simulink model "tennode_3"  (R2018b)
settings: Solver=ode3  StartTime=0.0  StopTime=5  FixedStep=Ts  RelTol=1e-3
values from neighbouring files (symbols this model uses):
  BESS_mode = 0    [load_vars.m]
  line1 = line1_length*R1    (= 0.01273)    [load_vars.m]
  line10 = line10_length*R1    (= 0.01273)    [load_vars.m]
  LINE10_en = 1    [load_vars.m]
  line11 = line11_length*R1    (= 0.01273)    [load_vars.m]
  LINE11_en = 1    [load_vars.m]
  line12 = line12_length*R1    (= 0.02546)    [load_vars.m]
  LINE12_en = 1    [load_vars.m]
  line13 = line13_length*R1    (= 0.015276)    [load_vars.m]
  LINE13_en = 1    [load_vars.m]
  line14 = line14_length*R1    (= 0.019095)    [load_vars.m]
  LINE14_en = 1    [load_vars.m]
  line15 = line15_length*R1    (= 0.014003)    [load_vars.m]
  LINE15_en = 1    [load_vars.m]
  line16 = line16_length*R1    (= 0.034371)    [load_vars.m]
  LINE16_en = 1    [load_vars.m]
  line17 = line17_length*R1    (= 0.017822)    [load_vars.m]
  LINE17_en = 1    [load_vars.m]
  LINE1_en = 1    [load_vars.m]
  line2 = line2_length*R1    (= 0.02546)    [load_vars.m]
  LINE2_en = 1    [load_vars.m]
  line3 = line3_length*R1    (= 0.015276)    [load_vars.m]
  LINE3_en = 1    [load_vars.m]
  line4 = line4_length*R1    (= 0.019095)    [load_vars.m]
  LINE4_en = 1    [load_vars.m]
  line5 = line5_length*R1    (= 0.014003)    [load_vars.m]
  LINE5_en = 1    [load_vars.m]
  line6 = line6_length*R1    (= 0.01273)    [load_vars.m]
  LINE6_en = 1    [load_vars.m]
  line7 = line7_length*R1    (= 0.03819)    [load_vars.m]
  LINE7_en = 1    [load_vars.m]
  line8 = line8_length*R1    (= 0.01273)    [load_vars.m]
  LINE8_en = 1    [load_vars.m]
  line9 = line9_length*R1    (= 0.01273)    [load_vars.m]
  LINE9_en = 1    [load_vars.m]
  t_contingency = 1    [load_vars.m]
  Ts = 0.0001    [load_vars.m]
  uDemand1 = 20e3    (= 20000)    [load_vars.m]
  uDemand10 = 20e3    (= 20000)    [load_vars.m]
  uDemand2 = 20e3    (= 20000)    [load_vars.m]
  uDemand3 = 20e3    (= 20000)    [load_vars.m]
  uDemand4 = 20e3    (= 20000)    [load_vars.m]
  uDemand5 = 20e3    (= 20000)    [load_vars.m]
  uDemand6 = 20e3    (= 20000)    [load_vars.m]
  uDemand7 = 20e3    (= 20000)    [load_vars.m]
  uDemand8 = 20e3    (= 20000)    [load_vars.m]
  uDemand9 = 20e3    (= 20000)    [load_vars.m]
undefined symbols (not defined in the file or in its folder): DER10_BESS_en, DER1_BESS_en, DER2_BESS_en, DER3_BESS_en, DER4_BESS_en, DER5_BESS_en, DER6_BESS_en, DER7_BESS_en, DER8_BESS_en, DER9_BESS_en, DR_capacity_1, DR_capacity_10, DR_capacity_2, DR_capacity_3, DR_capacity_4, DR_capacity_5, DR_capacity_6, DR_capacity_7, DR_capacity_8, DR_capacity_9, P_set1, P_set10, P_set2, P_set3, P_set4, P_set5, P_set6, P_set7, P_set8, P_set9, PV_capacity_1, PV_capacity_10, PV_capacity_2, PV_capacity_3, PV_capacity_4, PV_capacity_5, PV_capacity_6, PV_capacity_7, PV_capacity_8, PV_capacity_9, PV_en_1, PV_en_10, PV_en_2, PV_en_3, PV_en_4, PV_en_5, PV_en_6, PV_en_7, PV_en_8, PV_en_9
libraries: powerlib x232, simulink x66, powerlib_meascontrol x23, sps_avr x1, spsDieselMotorModel x1
(part 1 of 7)
settings Model: Creator=jjcla  LastModifiedBy=jjcla
settings SolverCC: ConcurrentTasks=on  AutoInsertRateTranBlk=on

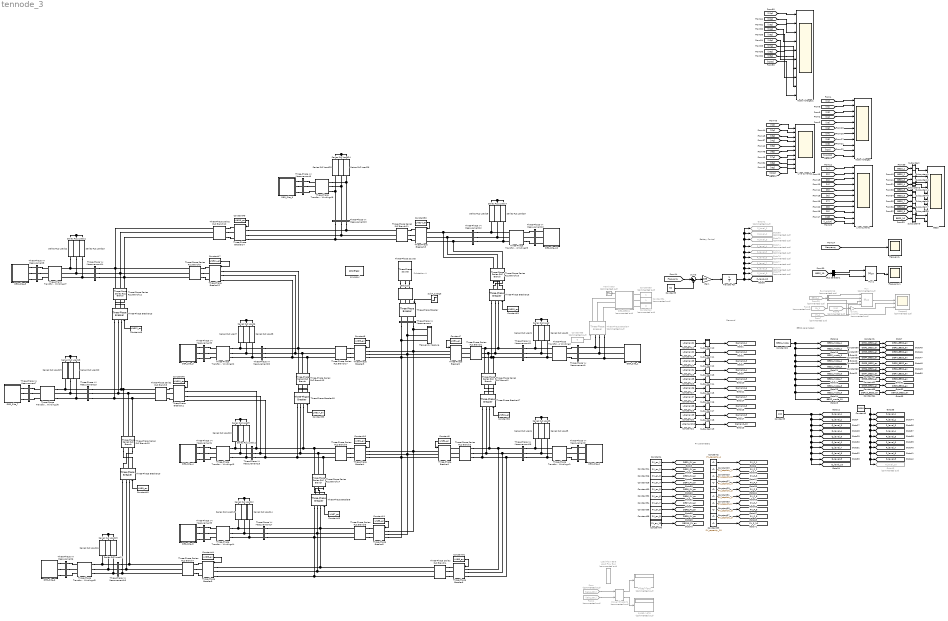
== system tennode_3 ==
  note: Substation A
  note: Battery Control
  note: Demand
  note: BESS parameters
  note: PV parameters
  66k/22k : powerlib/Elements/Three-Phase Transformer (Two Windings)  Winding1Connection=Yg  Winding2Connection=Y  CoreType=Three single-phase transformers  SetSaturation=off  Hysteresis=off  DataFile='hysteresis'  SetInitialFlux=off  Measurements=None  UNITS=pu  NominalPower=[ 10e6 , 50 ]  Winding1=[ 66e3 , 0.002 , 0.08 ]  Winding2=[22e3 , 0.002 , 0.08 ]  Rm=500  Lm=500  L0=0.5  Saturation=[ 0,0 ; 0.0024,1.2 ; 1.0,1.52 ]  InitialFluxes=[ 0.8 , -0.8 , 0.7 ]  MoreParameters=off  BreakLoop=on  DataType=off  TransfoNumber=1
      settings: SourceProductName=Simscape Electrical
  BESS : Scope  NumInputPorts=10
  Bus Selector1 : BusSelector  OutputSignals=Pbatt,Qbatt
  Bus Selector16 : BusSelector  Commented=on  OutputSignals=Pbatt,Qbatt,SOC (%)
  Constant1 : Constant  Value=DER1_BESS_en
  Constant10 : Constant  Value=LINE4_en
  Constant11 : Constant  Value=LINE5_en
  Constant12 : Constant  Value=uDemand1
  Constant13 : Constant  Value=uDemand2
  Constant14 : Constant  Value=uDemand3
  Constant15 : Constant  Value=uDemand4
  Constant16 : Constant  Value=uDemand5
  Constant17 : Constant  Value=uDemand6
  Constant18 : Constant  Value=uDemand7
  Constant19 : Constant  Value=uDemand8
  Constant2 : Constant  Value=PV_capacity_1
  Constant20 : Constant  Value=uDemand9
  Constant21 : Constant  Value=uDemand10
  Constant22 : Constant  Value=BESS_mode
  Constant23 : Constant  Value=PV_capacity_2
  Constant24 : Constant  Value=PV_en_2
  Constant25 : Constant  Value=PV_capacity_3
  Constant26 : Constant  Value=PV_en_3
  Constant27 : Constant  Value=PV_capacity_4
  Constant28 : Constant  Value=PV_en_4
  Constant29 : Constant  Value=PV_capacity_5
  Constant3 : Constant  Value=LINE2_en
  Constant30 : Constant  Value=PV_en_5
  Constant31 : Constant  Value=PV_capacity_6
  Constant32 : Constant  Value=PV_en_6
  Constant33 : Constant  Value=PV_capacity_7
  Constant34 : Constant  Value=PV_en_7
  Constant35 : Constant  Value=PV_capacity_8
  Constant36 : Constant  Value=PV_en_8
  Constant37 : Constant  Value=PV_capacity_9
  Constant38 : Constant  Value=PV_en_9
  Constant39 : Constant  Value=PV_capacity_10
  Constant4 : Constant  Value=PV_en_1
  Constant40 : Constant  Value=PV_en_10
  Constant41 : Constant  Value=LINE6_en
  Constant42 : Constant  Commented=on  Value=0
  Constant43 : Constant  Value=LINE7_en
  Constant44 : Constant  Value=LINE8_en
  Constant45 : Constant  Value=LINE9_en
  Constant46 : Constant  Value=LINE10_en
  Constant47 : Constant  Value=LINE11_en
  Constant48 : Constant  Value=LINE12_en
  Constant49 : Constant  Value=LINE13_en
  Constant5 : Constant  Value=100
  Constant50 : Constant  Value=LINE14_en
  Constant51 : Constant  Value=LINE15_en
  Constant52 : Constant  Value=LINE16_en
  Constant53 : Constant  Value=LINE17_en
  Constant54 : Constant  Commented=on
  Constant55 : Constant  Commented=on
  Constant56 : Constant  Value=DER2_BESS_en
  Constant57 : Constant  Value=DER3_BESS_en
  Constant58 : Constant  Value=DER4_BESS_en
  Constant59 : Constant  Value=DER5_BESS_en
  Constant6 : Constant  Value=5000
  Constant60 : Constant  Value=DER6_BESS_en
  Constant61 : Constant  Value=DER7_BESS_en
  Constant62 : Constant  Value=DER8_BESS_en
  Constant63 : Constant  Value=DER9_BESS_en
  Constant64 : Constant  Value=DER10_BESS_en
  Constant65 : Constant  Commented=on  Value=0
  Constant7 : Constant  Value=LINE1_en
  Constant8 : Constant  Value=LINE3_en
  Constant9 : Constant  Value=50
  DER_BESS1 : Subsystem  Commented=on  AncestorBlock=|  mask(Grid-connected Energy Storage (PQ Model)){SimMode=Electromagnetic Transient (EMT), Vn=400, Fn=50, PnomkW=5, kWh_Rated=13.5, Efficiency=96, LimitVec=[90 10], RechargeSOC=90, Precharge=50, autoRecharge=on, Initial_kWh_pc=80, PQvec=[500e3 0]}
      | microgridLibrary1/Energy Storage
      | (PQ Model)
      mask prompts: SimMode "Simulation Mode"; Vn "Nominal L-L Voltage [Vrms]"; Fn "Nominal Frequency [Hz]"; PnomkW "Rated Power [kW]"; kWh_Rated "Rated Capacity [kWh]"; Efficiency "Overall System Efficiency [%]"; LimitVec "Upper/Lower Charge Limits [%]"; RechargeSOC "SOC to Recharge [%]"; Precharge "Recharge Rate [% of Rated Power]"; autoRecharge "Enable Auto-Recharge"; Initial_kWh_pc "Initial State-of-Charge [0-100%]"; PQvec "Initial Active/Reactive Cmds"
      mask help:
      | The energy storage block models a generic grid-connected energy storage system (ESS), most commonly a battery system. This is a system-level model that does not contain any power electronics, but is useful for load flow, phasor, and hybrid phasor-EMT simulations. The inputs to this block are the commanded active and reactive power of the ESS. The ESS is assumed to have four quadrent operation. The Mode Input dictates what high-level operation the ESS has: current control (Mode = 1) or voltage control (Mode = 0). Current control is ideal for a grid connected system where you need to specify P,Q commands. Voltage control is necessary if the ESS will be the only system supporting the microgrid in islanded mode.
      |
      | For more detailed ESS models, consider the battery block in the Drives library. Consider using this PQ Model to perform load flow studies and switch to a more detailed model when full EMT studies or more advanced controls are required.
      |
      | Note: The initial active/reactive power commands must be specified for use for Load Flow analysis.
      mask init:
      | % Calculate Initial Conditions
      | Pnom = PnomkW*1e3;
      | P0 = -PQvec(1);  Q0 = -PQvec(2);
      | if abs(P0) > Pnom
      |     P0 = sign(P0)*Pnom;
      | end
      | 
      | % Calculate Q0 given Reactive Power Capability Curve
      | Qlim = sqrt(Pnom^2 - P0^2);
      | if Qlim > abs(Q0)
      |     Q0 = sign(Q0)*Qlim;
      | end
      | 
      | UpChrgLim = LimitVec(1);
      | LowChrgLim = LimitVec(2);
      | if Initial_kWh_pc > UpChrgLim && P0 < 0
      |     P0 = 0; Q0 = 0;
      | elseif Initial_kWh_pc < LowChrgLim && P0 > 0
      |     P0 = 0; Q0 = 0;
      | end
      | 
      | simulationStatus =  get_param(bdroot,'SimulationStatus');
      | 
      | % The active variant can only be modified at edit-time or very early during
      | % the simulink compile stage. 
      | if any(strcmp(simulationStatus, {'stopped'}))
      | 
      | blk = [gcb '/Power Measures'];
      | if strcmp(SimMode,'Phasor')
      |     set_param(blk,'OverrideUsingVariant','Phasor');
      | else
      |     set_param(blk,'OverrideUsingVariant','EMT');
      | end
      | 
      | 
      | end
      mask TypeOptions SimMode: Electromagnetic Transient (EMT) | Phasor
      mask DialogControl Container7 Prompt: Grid Connection Properties
      mask DialogControl Container11 Prompt: Charge/Discharge Controls
      mask DialogControl Container12 Prompt: Initial Conditions
      mask Display: plot(-80,-50,80,50,[0,9,18,24,29,30,29,24,18,9,0,-9,-18,-24,-29,-30,-29,-24,-18,-9,0],[30,29,24,18,9,0,-9,-18,-24,-29,-30,-29,-24,-18,-9,0,9,18,24,29,30],[-50],[0],[50],[0],[45 35 40 40 40],[15 15 15 20 10],[1 2 3 4 5 6 7 8 9 10 11 12 13 14 15 16 17 18 19 20 21].*1.5-15,[0,9,18,24,29,30,29,24,18,9,0,-9,-18,-24,-29,-30,-29,-24,-18,-9,0]./2.4)
  DER_Site_1 : Subsystem
  DER_Site_10 : Subsystem
  DER_Site_2 : Subsystem
  DER_Site_3 : Subsystem
  DER_Site_4 : Subsystem
  DER_Site_5 : Subsystem
  DER_Site_6 : Subsystem
  DER_Site_7 : Subsystem
  DER_Site_8 : Subsystem
  DER_Site_9 : Subsystem
  Frequency : Scope
  Frequency Measure : Subsystem
  Frequency1 : Scope
  From : From  Commented=on  GotoTag=Vabc_001  TagVisibility=global
  From1 : From  Commented=on  GotoTag=Iabc_001  TagVisibility=global
  From25 : From  Commented=on  GotoTag=BESS_1  TagVisibility=global
  From6 : From  Commented=on  GotoTag=V1  TagVisibility=global
  From7 : From  Commented=on  GotoTag=PV_1  TagVisibility=global
  From8 : From  Commented=on  GotoTag=SL_1  TagVisibility=global
  Gain : Gain  Gain=1e5
  Goto43 : Goto  Commented=on  GotoTag=P_level_10  TagVisibility=global
  Goto72 : Goto  Commented=on  GotoTag=P_level_1  TagVisibility=global
  Goto73 : Goto  Commented=on  GotoTag=P_level_3  TagVisibility=global
  Goto74 : Goto  Commented=on  GotoTag=P_level_4  TagVisibility=global
  Goto75 : Goto  Commented=on  GotoTag=P_level_5  TagVisibility=global
  Goto76 : Goto  Commented=on  GotoTag=P_level_6  TagVisibility=global
  Goto77 : Goto  Commented=on  GotoTag=P_level_7  TagVisibility=global
  Goto78 : Goto  Commented=on  GotoTag=P_level_8  TagVisibility=global
  Goto79 : Goto  Commented=on  GotoTag=P_level_9  TagVisibility=global
  Goto80 : Goto  Commented=on  GotoTag=P_level_2  TagVisibility=global
  Line Currents : Scope  NumInputPorts=11
  Line Currents1 : Scope  NumInputPorts=10
  Load Flow Bar6 : powerlib/Measurements/Load Flow Bus  Commented=on  LConnTagsString=a|b|c  RConnTagsString=a|b|c  Phases=ABC  Connectors=on both sides  ID=001  Vbase=22000/sqrt(3)  Vref=[1.0 1.0 1.0]  Vangle=[0 -120 120]  VLF=0.9871  VLFb=1.052  VLFc=0.978  angleLF=-5.528  angleLFb=-122.4  angleLFc=116
      settings: AttributesFormatString=%<ID>  SourceProductName=Simscape Electrical
  Mux : Mux  Commented=on
      settings: DisplayOption=signals
  Mux1 : Mux  Inputs=2
      settings: DisplayOption=signals
  Node Voltages : Scope  NumInputPorts=11
  Node Voltages1 : Scope  NumInputPorts=10
  P 692->675 : Display  Commented=on
  Power (Phasor)1 : powerlib_meascontrol/Measurements/Power (Phasor)  Commented=on
      settings: SourceProductName=Simscape Electrical  SourceProductBaseCode=PS
  Q 692->675 : Display  Commented=on
  Scopes1 : Scope  Commented=on  NumInputPorts=4
  Series RLC Load{,1..29} (30 alike) : powerlib/Elements/Series RLC Load  LConnTagsString=a  RConnTagsString=__new0  NominalVoltage=22e3  NominalFrequency=50  ActivePower=10e3  InductivePower=100  CapacitivePower=100  Setx0=off  InitialVoltage=0  SetiL0=off  InitialCurrent=0  Measurements=None  LoadType=constant Z
      settings: SourceProductName=Simscape Electrical
  SubA_outage : Step  Time=t_contingency  Before=1  After=0  SampleTime=0
  Subsystem : Subsystem
  Subsystem1 : Subsystem
  Subsystem10 : Subsystem
  Subsystem11 : Subsystem
  Subsystem12 : Subsystem
  Subsystem13 : Subsystem
  Subsystem14 : Subsystem
  Subsystem15 : Subsystem
  Subsystem16 : Subsystem
  Subsystem17 : Subsystem
  Subsystem18 : Subsystem
  Subsystem19 : Subsystem
  Subsystem2 : Subsystem
  Subsystem3 : Subsystem
  Subsystem4 : Subsystem
  Subsystem5 : Subsystem
  Subsystem6 : Subsystem
  Subsystem7 : Subsystem
  Subsystem8 : Subsystem
  Subsystem9 : Subsystem
  Sum3 : Sum  Inputs=|+-
  Terminator : Terminator  Commented=on
  Three-Phase Series RLC Branch1 : powerlib/Elements/Three-Phase Series RLC Branch  LConnTagsString=A|B|C  RConnTagsString=A|B|C  BranchType=R  Resistance=line1  Inductance=10e-6  Capacitance=10e-9  Measurements=Branch currents
  Three-Phase Series RLC Branch10 : powerlib/Elements/Three-Phase Series RLC Branch  LConnTagsString=A|B|C  RConnTagsString=A|B|C  BranchType=R  Resistance=line13  Inductance=10e-6  Capacitance=10e-9  Measurements=Branch currents
  Three-Phase Series RLC Branch11 : powerlib/Elements/Three-Phase Series RLC Branch  LConnTagsString=A|B|C  RConnTagsString=A|B|C  BranchType=R  Resistance=line14  Inductance=10e-6  Capacitance=10e-9  Measurements=Branch currents
  Three-Phase Series RLC Branch12 : powerlib/Elements/Three-Phase Series RLC Branch  LConnTagsString=A|B|C  RConnTagsString=A|B|C  BranchType=R  Resistance=line12  Inductance=10e-6  Capacitance=10e-9  Measurements=Branch currents
  Three-Phase Series RLC Branch13 : powerlib/Elements/Three-Phase Series RLC Branch  LConnTagsString=A|B|C  RConnTagsString=A|B|C  BranchType=R  Resistance=line17  Inductance=10e-6  Capacitance=10e-9  Measurements=Branch currents
  Three-Phase Series RLC Branch14 : powerlib/Elements/Three-Phase Series RLC Branch  LConnTagsString=A|B|C  RConnTagsString=A|B|C  BranchType=R  Resistance=line7  Inductance=10e-6  Capacitance=10e-9  Measurements=Branch currents
  Three-Phase Series RLC Branch15 : powerlib/Elements/Three-Phase Series RLC Branch  LConnTagsString=A|B|C  RConnTagsString=A|B|C  BranchType=R  Resistance=line9  Inductance=10e-6  Capacitance=10e-9  Measurements=Branch currents
  Three-Phase Series RLC Branch16 : powerlib/Elements/Three-Phase Series RLC Branch  LConnTagsString=A|B|C  RConnTagsString=A|B|C  BranchType=R  Resistance=line15  Inductance=10e-6  Capacitance=10e-9  Measurements=Branch currents
  Three-Phase Series RLC Branch17 : powerlib/Elements/Three-Phase Series RLC Branch  LConnTagsString=A|B|C  RConnTagsString=A|B|C  BranchType=R  Resistance=line3  Inductance=10e-6  Capacitance=10e-9  Measurements=Branch currents
  Three-Phase Series RLC Branch2 : powerlib/Elements/Three-Phase Series RLC Branch  LConnTagsString=A|B|C  RConnTagsString=A|B|C  BranchType=R  Resistance=line16  Inductance=10e-6  Capacitance=10e-9  Measurements=Branch currents
  Three-Phase Series RLC Branch3 : powerlib/Elements/Three-Phase Series RLC Branch  LConnTagsString=A|B|C  RConnTagsString=A|B|C  BranchType=R  Resistance=line2  Inductance=10e-6  Capacitance=10e-9  Measurements=Branch currents
  Three-Phase Series RLC Branch4 : powerlib/Elements/Three-Phase Series RLC Branch  LConnTagsString=A|B|C  RConnTagsString=A|B|C  BranchType=R  Resistance=line6  Inductance=10e-6  Capacitance=10e-9  Measurements=Branch currents
  Three-Phase Series RLC Branch5 : powerlib/Elements/Three-Phase Series RLC Branch  LConnTagsString=A|B|C  RConnTagsString=A|B|C  BranchType=R  Resistance=line5  Inductance=10e-6  Capacitance=10e-9  Measurements=Branch currents
  Three-Phase Series RLC Branch6 : powerlib/Elements/Three-Phase Series RLC Branch  LConnTagsString=A|B|C  RConnTagsString=A|B|C  BranchType=R  Resistance=line4  Inductance=10e-6  Capacitance=10e-9  Measurements=Branch currents
  Three-Phase Series RLC Branch7 : powerlib/Elements/Three-Phase Series RLC Branch  LConnTagsString=A|B|C  RConnTagsString=A|B|C  BranchType=R  Resistance=line8  Inductance=10e-6  Capacitance=10e-9  Measurements=Branch currents
  Three-Phase Series RLC Branch8 : powerlib/Elements/Three-Phase Series RLC Branch  LConnTagsString=A|B|C  RConnTagsString=A|B|C  BranchType=R  Resistance=line10  Inductance=10e-6  Capacitance=10e-9  Measurements=Branch currents
  Three-Phase Series RLC Branch9 : powerlib/Elements/Three-Phase Series RLC Branch  LConnTagsString=A|B|C  RConnTagsString=A|B|C  BranchType=R  Resistance=line11  Inductance=10e-6  Capacitance=10e-9  Measurements=Branch currents
  Three-Phase Source : powerlib/Electrical Sources/Three-Phase Source  InternalConnection=Yg  VoltagePhases=off  Voltage=66e3  PhaseAngle=0  Voltage_phases=[25e3 25e3 25e3]/sqrt(3)  PhaseAngles_phases=[0 -120 +120]  Frequency=50  NonIdealSource=on  SpecifyImpedance=on  Resistance=0.8929  Inductance=16.58e-3  ShortCircuitLevel=100e6  BaseVoltage=25e3  XRratio=7  BusType=swing  Pref=0  Qref=0  Prefabc=[10e3, 10e3, 10e3]  Qrefabc=[0, 0, 0]  Qmin=-inf  Qmax=inf
      settings: SourceProductName=Simscape Electrical
  Three-Phase Transformer (Two Windings){,1..9} (10 alike) : powerlib/Elements/Three-Phase Transformer (Two Windings)  Winding1Connection=Yg  Winding2Connection=Yg  CoreType=Three single-phase transformers  SetSaturation=off  Hysteresis=off  DataFile='hysteresis'  SetInitialFlux=off  Measurements=None  UNITS=pu  NominalPower=[ 250e6 , 50 ]  Winding1=[ 22e3 , 0.002 , 0.08 ]  Winding2=[ 400 , 0.002 , 0.08 ]  Rm=500  Lm=500  L0=0.5  Saturation=[ 0,0 ; 0.0024,1.2 ; 1.0,1.52 ]  InitialFluxes=[ 0.8 , -0.8 , 0.7 ]  MoreParameters=off  BreakLoop=off  DataType=off  TransfoNumber=1
      settings: SourceProductName=Simscape Electrical
  Three-Phase V-I Measurement : powerlib/Measurements/Three-Phase V-I Measurement  VoltageMeasurement=phase-to-ground  SetLabelV=on  LabelV=V_subA  Vpu=off  VpuLL=off  CurrentMeasurement=yes  SetLabelI=on  LabelI=I_subA  Ipu=off  Pbase=100e6  Vbase=500e3  OutputType=Complex  PhasorSimulation=on  PSBequivalent=0
      settings: SourceProductName=Simscape Electrical
  Three-Phase V-I Measurement1 : powerlib/Measurements/Three-Phase V-I Measurement  VoltageMeasurement=phase-to-phase  SetLabelV=on  LabelV=V1  Vpu=off  VpuLL=off  CurrentMeasurement=yes  SetLabelI=on  LabelI=I1  Ipu=off  Pbase=100e6  Vbase=500e3  OutputType=Complex  PhasorSimulation=off  PSBequivalent=0
      settings: SourceProductName=Simscape Electrical
  Three-Phase V-I Measurement10 : powerlib/Measurements/Three-Phase V-I Measurement  VoltageMeasurement=phase-to-phase  SetLabelV=on  LabelV=V10  Vpu=off  VpuLL=off  CurrentMeasurement=yes  SetLabelI=on  LabelI=I10  Ipu=off  Pbase=100e6  Vbase=500e3  OutputType=Complex  PhasorSimulation=off  PSBequivalent=0
      settings: SourceProductName=Simscape Electrical
  Three-Phase V-I Measurement11 : powerlib/Measurements/Three-Phase V-I Measurement  VoltageMeasurement=phase-to-phase  SetLabelV=on  LabelV=V1p  Vpu=off  VpuLL=off  CurrentMeasurement=yes  SetLabelI=on  LabelI=I1p  Ipu=off  Pbase=100e6  Vbase=500e3  OutputType=Complex  PhasorSimulation=off  PSBequivalent=0
      settings: SourceProductName=Simscape Electrical
  Three-Phase V-I Measurement12 : powerlib/Measurements/Three-Phase V-I Measurement  VoltageMeasurement=phase-to-phase  SetLabelV=on  LabelV=V10p  Vpu=off  VpuLL=off  CurrentMeasurement=yes  SetLabelI=on  LabelI=I10p  Ipu=off  Pbase=100e6  Vbase=500e3  OutputType=Complex  PhasorSimulation=off  PSBequivalent=0
      settings: SourceProductName=Simscape Electrical
  Three-Phase V-I Measurement13 : powerlib/Measurements/Three-Phase V-I Measurement  VoltageMeasurement=phase-to-phase  SetLabelV=on  LabelV=V9p  Vpu=off  VpuLL=off  CurrentMeasurement=yes  SetLabelI=on  LabelI=I9p  Ipu=off  Pbase=100e6  Vbase=500e3  OutputType=Complex  PhasorSimulation=off  PSBequivalent=0
      settings: SourceProductName=Simscape Electrical
  Three-Phase V-I Measurement14 : powerlib/Measurements/Three-Phase V-I Measurement  VoltageMeasurement=phase-to-phase  SetLabelV=on  LabelV=V8p  Vpu=off  VpuLL=off  CurrentMeasurement=yes  SetLabelI=on  LabelI=I8p  Ipu=off  Pbase=100e6  Vbase=500e3  OutputType=Complex  PhasorSimulation=off  PSBequivalent=0
      settings: SourceProductName=Simscape Electrical
  Three-Phase V-I Measurement15 : powerlib/Measurements/Three-Phase V-I Measurement  VoltageMeasurement=phase-to-phase  SetLabelV=on  LabelV=V7p  Vpu=off  VpuLL=off  CurrentMeasurement=yes  SetLabelI=on  LabelI=I7p  Ipu=off  Pbase=100e6  Vbase=500e3  OutputType=Complex  PhasorSimulation=off  PSBequivalent=0
      settings: SourceProductName=Simscape Electrical
  Three-Phase V-I Measurement16 : powerlib/Measurements/Three-Phase V-I Measurement  VoltageMeasurement=phase-to-phase  SetLabelV=on  LabelV=V6p  Vpu=off  VpuLL=off  CurrentMeasurement=yes  SetLabelI=on  LabelI=I6p  Ipu=off  Pbase=100e6  Vbase=500e3  OutputType=Complex  PhasorSimulation=off  PSBequivalent=0
      settings: SourceProductName=Simscape Electrical
  Three-Phase V-I Measurement17 : powerlib/Measurements/Three-Phase V-I Measurement  VoltageMeasurement=phase-to-phase  SetLabelV=on  LabelV=V5p  Vpu=off  VpuLL=off  CurrentMeasurement=yes  SetLabelI=on  LabelI=I5p  Ipu=off  Pbase=100e6  Vbase=500e3  OutputType=Complex  PhasorSimulation=off  PSBequivalent=0
      settings: SourceProductName=Simscape Electrical
  Three-Phase V-I Measurement18 : powerlib/Measurements/Three-Phase V-I Measurement  VoltageMeasurement=phase-to-phase  SetLabelV=on  LabelV=V2p  Vpu=off  VpuLL=off  CurrentMeasurement=yes  SetLabelI=on  LabelI=I2p  Ipu=off  Pbase=100e6  Vbase=500e3  OutputType=Complex  PhasorSimulation=off  PSBequivalent=0
      settings: SourceProductName=Simscape Electrical
  Three-Phase V-I Measurement19 : powerlib/Measurements/Three-Phase V-I Measurement  VoltageMeasurement=phase-to-phase  SetLabelV=on  LabelV=V4p  Vpu=off  VpuLL=off  CurrentMeasurement=yes  SetLabelI=on  LabelI=I4p  Ipu=off  Pbase=100e6  Vbase=500e3  OutputType=Complex  PhasorSimulation=off  PSBequivalent=0
      settings: SourceProductName=Simscape Electrical
  Three-Phase V-I Measurement2 : powerlib/Measurements/Three-Phase V-I Measurement  VoltageMeasurement=phase-to-phase  SetLabelV=on  LabelV=V2  Vpu=off  VpuLL=off  CurrentMeasurement=yes  SetLabelI=on  LabelI=I2  Ipu=off  Pbase=100e6  Vbase=500e3  OutputType=Complex  PhasorSimulation=off  PSBequivalent=0
      settings: SourceProductName=Simscape Electrical
  Three-Phase V-I Measurement20 : powerlib/Measurements/Three-Phase V-I Measurement  VoltageMeasurement=phase-to-phase  SetLabelV=on  LabelV=V3p  Vpu=off  VpuLL=off  CurrentMeasurement=yes  SetLabelI=on  LabelI=I3p  Ipu=off  Pbase=100e6  Vbase=500e3  OutputType=Complex  PhasorSimulation=off  PSBequivalent=0
      settings: SourceProductName=Simscape Electrical
  Three-Phase V-I Measurement3 : powerlib/Measurements/Three-Phase V-I Measurement  VoltageMeasurement=phase-to-phase  SetLabelV=on  LabelV=V3  Vpu=off  VpuLL=off  CurrentMeasurement=yes  SetLabelI=on  LabelI=I3  Ipu=off  Pbase=100e6  Vbase=500e3  OutputType=Complex  PhasorSimulation=off  PSBequivalent=0
      settings: SourceProductName=Simscape Electrical
  Three-Phase V-I Measurement4 : powerlib/Measurements/Three-Phase V-I Measurement  VoltageMeasurement=phase-to-phase  SetLabelV=on  LabelV=V4  Vpu=off  VpuLL=off  CurrentMeasurement=yes  SetLabelI=on  LabelI=I4  Ipu=off  Pbase=100e6  Vbase=500e3  OutputType=Complex  PhasorSimulation=off  PSBequivalent=0
      settings: SourceProductName=Simscape Electrical
  Three-Phase V-I Measurement5 : powerlib/Measurements/Three-Phase V-I Measurement  VoltageMeasurement=phase-to-phase  SetLabelV=on  LabelV=V5  Vpu=off  VpuLL=off  CurrentMeasurement=yes  SetLabelI=on  LabelI=I5  Ipu=off  Pbase=100e6  Vbase=500e3  OutputType=Complex  PhasorSimulation=off  PSBequivalent=0
      settings: SourceProductName=Simscape Electrical
  Three-Phase V-I Measurement6 : powerlib/Measurements/Three-Phase V-I Measurement  VoltageMeasurement=phase-to-phase  SetLabelV=on  LabelV=V6  Vpu=off  VpuLL=off  CurrentMeasurement=yes  SetLabelI=on  LabelI=I6  Ipu=off  Pbase=100e6  Vbase=500e3  OutputType=Complex  PhasorSimulation=off  PSBequivalent=0
      settings: SourceProductName=Simscape Electrical
  Three-Phase V-I Measurement7 : powerlib/Measurements/Three-Phase V-I Measurement  VoltageMeasurement=phase-to-phase  SetLabelV=on  LabelV=V7  Vpu=off  VpuLL=off  CurrentMeasurement=yes  SetLabelI=on  LabelI=I7  Ipu=off  Pbase=100e6  Vbase=500e3  OutputType=Complex  PhasorSimulation=off  PSBequivalent=0
      settings: SourceProductName=Simscape Electrical
  Three-Phase V-I Measurement8 : powerlib/Measurements/Three-Phase V-I Measurement  VoltageMeasurement=phase-to-phase  SetLabelV=on  LabelV=V8  Vpu=off  VpuLL=off  CurrentMeasurement=yes  SetLabelI=on  LabelI=I8  Ipu=off  Pbase=100e6  Vbase=500e3  OutputType=Complex  PhasorSimulation=off  PSBequivalent=0
      settings: SourceProductName=Simscape Electrical
  Three-Phase V-I Measurement9 : powerlib/Measurements/Three-Phase V-I Measurement  VoltageMeasurement=phase-to-phase  SetLabelV=on  LabelV=V9  Vpu=off  VpuLL=off  CurrentMeasurement=yes  SetLabelI=on  LabelI=I9  Ipu=off  Pbase=100e6  Vbase=500e3  OutputType=Complex  PhasorSimulation=off  PSBequivalent=0
      settings: SourceProductName=Simscape Electrical
  Three-Phase Breaker{,1..6,8..18} (18 alike) : powerlib/Elements/Three-Phase Breaker  InitialState=closed  SwitchA=on  SwitchB=on  SwitchC=on  SwitchTimes="[1/60  5/60]"  External=on  BreakerResistance=0.01  SnubberResistance=1e6  SnubberCapacitance=inf  Measurements=None
      settings: SourceProductName=Simscape Electrical
  Three-Phase Breaker7 : powerlib/Elements/Three-Phase Breaker  Commented=on  InitialState=open  SwitchA=on  SwitchB=on  SwitchC=on  SwitchTimes="[1/60  5/60]"  External=on  BreakerResistance=0.01  SnubberResistance=1e6  SnubberCapacitance=inf  Measurements=None
      settings: SourceProductName=Simscape Electrical
  Transfer Fcn : TransferFcn  Denominator=[1 0]
  powergui : powerlib/powergui  Priority=1  SimulationMode=Discrete  SampleTime=Ts  frequency=60  Iterations=50  frequencyindice=0  Pbase=100e6  ErrMax=0.0001  UnitsV=kV  UnitsW=MW  buscounter=3  FunctionMessages=off  echomessages=off  EnableUseOfTLC=off  CurrentSourceSwitches=off  DisableSnubberDevices=off  DisableRonSwitches=off  DisableVfSwitches=off  DisplayEquations=off  SolverType=Tustin/Backward Euler (TBE)  Interpol=off  ExternalGateDelay=off  methode=off  Ts=100  x0status=blocks  SPID=on  SwTol=0  HookPort=off  RestoreLinks=warning  ResistiveCurrentMeasurement=off  Frange=[0:2:500]  Ylog=off  Xlog=on  ShowGrid=off  save=off  variable=ZData  structure=0  ZoomFFT=off  StartTime=0.0  cycles=1  DisplayStyle=1  fundamental=60  FreqAxis=off  MaxFrequency=1000  frequencyindicesteady=1  RmsSteady=1  display=off
  to kW1 : Gain  Commented=on  Gain=1/sqrt(2)
  tag scope: BESS_mode_10=global, BESS_mode_1=global, BESS_mode_2=global, BESS_mode_3=global, BESS_mode_4=global, BESS_mode_5=global, BESS_mode_6=global, BESS_mode_7=global, BESS_mode_8=global, BESS_mode_9=global, DER10_BESS_en=global, DER10_PV_en=global, DER1_BESS_en=global, DER1_PV_en=global, DER2_BESS_en=global, DER2_PV_en=global, DER3_BESS_en=global, DER3_PV_en=global, DER4_BESS_en=global, DER4_PV_en=global, DER5_BESS_en=global, DER5_PV_en=global, DER6_BESS_en=global, DER6_PV_en=global, DER7_BESS_en=global, DER7_PV_en=global, DER8_BESS_en=global, DER8_PV_en=global, DER9_BESS_en=global, DER9_PV_en=global, Demand_10=global, Demand_1=global, Demand_2=global, Demand_3=global, Demand_4=global, Demand_5=global, Demand_6=global, Demand_7=global, Demand_8=global, Demand_9=global, PV_P_10=global, PV_P_1=global, PV_P_2=global, PV_P_3=global, PV_P_4=global, PV_P_5=global, PV_P_6=global, PV_P_7=global, PV_P_8=global, PV_P_9=global, P_level_10=global, P_level_1=global, P_level_2=global, P_level_3=global, P_level_4=global, P_level_5=global, P_level_6=global, P_level_7=global, P_level_8=global, P_level_9=global, Q_level_10=global, Q_level_1=global, Q_level_2=global, Q_level_3=global, Q_level_4=global, Q_level_5=global, Q_level_6=global, Q_level_7=global, Q_level_8=global, Q_level_9=global
  wires:
  SubA_outage/1 -> Three-Phase Breaker/1
  From6/1 -> to kW1/1
  From25/1 -> Bus Selector16/1
  Constant1/1 -> [DER1_BESS_en]
  Constant2/1 -> [PV_P_1]
  Constant4/1 -> [DER1_PV_en]
  to kW1/1 -> Scopes1/3  "Voltage"
  Bus Selector16/2 -> Mux/2  "<Qbatt>"
  Bus Selector16/1 -> Mux/1  "<Pbatt>"
  Bus Selector16/3 -> Scopes1/4  "<SOC (%)>"
  Mux/1 -> Scopes1/2  "Power Output"
  From8/1 -> Mux/3
  From7/1 -> Mux/4  "PV Power"
  Constant7/1 -> Three-Phase Breaker2/1
  [Frequency] -> Sum3/1
  Constant9/1 -> Sum3/2
  Sum3/1 -> Gain/1
  Gain/1 -> Transfer Fcn/1
  Constant3/1 -> Three-Phase Breaker1/1
  Constant8/1 -> Three-Phase Breaker3/1
  Constant10/1 -> Three-Phase Breaker4/1
  Constant11/1 -> Three-Phase Breaker5/1
  Constant22/1 -> [BESS_mode_10], [BESS_mode_9], [BESS_mode_8], [BESS_mode_7], [BESS_mode_6], [BESS_mode_5], [BESS_mode_4], [BESS_mode_3], [BESS_mode_2], [BESS_mode_1]
  Constant5/1 -> [Q_level_2], [Q_level_3], [Q_level_5], [Q_level_6], [Q_level_7], [Q_level_8], [Q_level_9], [Q_level_10], [Q_level_4], [Q_level_1]
  Constant6/1 -> [P_level_3], [P_level_4], [P_level_6], [P_level_8], [P_level_9], Goto43/1, [P_level_7], [P_level_5], [P_level_2], [P_level_1]
  Constant23/1 -> [PV_P_2]
  Constant24/1 -> [DER2_PV_en]
  Constant25/1 -> [PV_P_3]
  Constant26/1 -> [DER3_PV_en]
  Constant27/1 -> [PV_P_4]
  Constant28/1 -> [DER4_PV_en]
  Constant29/1 -> [PV_P_5]
  Constant30/1 -> [DER5_PV_en]
  Constant32/1 -> [DER6_PV_en]
  Constant31/1 -> [PV_P_6]
  Constant34/1 -> [DER7_PV_en]
  Constant33/1 -> [PV_P_7]
  Constant36/1 -> [DER8_PV_en]
  Constant35/1 -> [PV_P_8]
  Constant38/1 -> [DER9_PV_en]
  Constant37/1 -> [PV_P_9]
  Constant40/1 -> [DER10_PV_en]
  Constant39/1 -> [PV_P_10]
  Constant41/1 -> Three-Phase Breaker6/1
  Constant43/1 -> Three-Phase Breaker8/1
  Constant44/1 -> Three-Phase Breaker9/1
  Constant45/1 -> Three-Phase Breaker10/1
  Constant46/1 -> Three-Phase Breaker11/1
  Constant47/1 -> Three-Phase Breaker12/1
  Constant48/1 -> Three-Phase Breaker13/1
  Constant49/1 -> Three-Phase Breaker14/1
  Constant50/1 -> Three-Phase Breaker15/1
  Constant51/1 -> Three-Phase Breaker16/1
  Constant52/1 -> Three-Phase Breaker17/1
  Constant53/1 -> Three-Phase Breaker18/1
  [Frequency] -> Frequency/1  "System_Frequency"
  Constant42/1 -> DER_BESS1/3(Mode)
  Constant55/1 -> DER_BESS1/1(Pref)
  Constant54/1 -> DER_BESS1/2(Qref)
  DER_BESS1/1(m) -> Terminator/1
  Constant58/1 -> [DER4_BESS_en]
  Constant59/1 -> [DER5_BESS_en]
  Constant62/1 -> [DER8_BESS_en]
  Constant63/1 -> [DER9_BESS_en]
  Constant64/1 -> [DER10_BESS_en]
  Constant61/1 -> [DER7_BESS_en]
  Constant60/1 -> [DER6_BESS_en]
  Constant57/1 -> [DER3_BESS_en]
  Constant56/1 -> [DER2_BESS_en]
  Constant12/1 -> Subsystem10/1(In1)
  Subsystem10/1(Out1) -> [Demand_1]
  Constant13/1 -> Subsystem11/1(In1)
  Subsystem11/1(Out1) -> [Demand_2]
  Constant14/1 -> Subsystem12/1(In1)
  Subsystem12/1(Out1) -> [Demand_3]
  Constant15/1 -> Subsystem13/1(In1)
  Subsystem13/1(Out1) -> [Demand_4]
  Constant16/1 -> Subsystem14/1(In1)
  Subsystem14/1(Out1) -> [Demand_5]
  Constant17/1 -> Subsystem15/1(In1)
  Constant18/1 -> Subsystem16/1(In1)
  Constant19/1 -> Subsystem17/1(In1)
  Constant20/1 -> Subsystem18/1(In1)
  Constant21/1 -> Subsystem19/1(In1)
  Subsystem15/1(Out1) -> [Demand_6]
  Subsystem16/1(Out1) -> [Demand_7]
  Subsystem17/1(Out1) -> [Demand_8]
  Subsystem18/1(Out1) -> [Demand_9]
  Subsystem19/1(Out1) -> [Demand_10]
  Power (Phasor)1/2 -> Q 692->675/1
  From/1 -> Power (Phasor)1/1
  From1/1 -> Power (Phasor)1/2
  Power (Phasor)1/1 -> P 692->675/1
  Constant65/1 -> Three-Phase Breaker7/1
  [I10] -> Line Currents/10
  [I1] -> Line Currents/1
  [I2] -> Line Currents/2
  [I3] -> Line Currents/3
  [I4] -> Line Currents/4
  [I5] -> Line Currents/5
  [I6] -> Line Currents/6
  [I7] -> Line Currents/7
  [I8] -> Line Currents/8
  [I9] -> Line Currents/9
  [I_subA] -> Line Currents/11
  [V1] -> Node Voltages/1
  [V2] -> Node Voltages/2
  [V3] -> Node Voltages/3
  [V4] -> Node Voltages/4
  [V5] -> Node Voltages/5
  [V6] -> Node Voltages/6
  [V7] -> Node Voltages/7
  [V8] -> Node Voltages/8
  [V9] -> Node Voltages/9
  [V10] -> Node Voltages/10
  [V_subA] -> Node Voltages/11
  Bus Selector1/1 -> Mux1/1  "<Pbatt>"
  Bus Selector1/2 -> Mux1/2  "<Qbatt>"
  [BESS_10] -> Bus Selector1/1
  Mux1/1 -> Frequency1/1  "Power Output"
  [BESS_9] -> Subsystem8/1(In1)
  [BESS_10] -> Subsystem9/1(In1)
  [BESS_5] -> Subsystem4/1(In1)
  [BESS_8] -> Subsystem7/1(In1)
  [BESS_6] -> Subsystem5/1(In1)
  [BESS_3] -> Subsystem2/1(In1)
  [BESS_2] -> Subsystem1/1(In1)
  [BESS_1] -> Subsystem/1(In1)
  [BESS_7] -> Subsystem6/1(In1)
  Subsystem/1(Power Output) -> BESS/1
  Subsystem1/1(Power Output) -> BESS/2
  Subsystem2/1(Power Output) -> BESS/3
  [BESS_4] -> Subsystem3/1(In1)
  Subsystem3/1(Power Output) -> BESS/4
  Subsystem4/1(Power Output) -> BESS/5
  Subsystem5/1(Power Output) -> BESS/6
  Subsystem6/1(Power Output) -> BESS/7
  Subsystem7/1(Power Output) -> BESS/8
  Subsystem8/1(Power Output) -> BESS/9
  Subsystem9/1(Power Output) -> BESS/10
  Transfer Fcn/1 -> Goto73/1, Goto80/1, Goto72/1, Goto74/1, Goto75/1, Goto76/1, Goto77/1, Goto78/1, Goto79/1, [P_level_10]
  [I10p] -> Line Currents1/10
  [I4p] -> Line Currents1/4
  [I2p] -> Line Currents1/2
  [I7p] -> Line Currents1/7
  [I9p] -> Line Currents1/9
  [I3p] -> Line Currents1/3
  [V4p] -> Node Voltages1/4
  [V9p] -> Node Voltages1/9
  [V10p] -> Node Voltages1/10
  [V5p] -> Node Voltages1/5
  [V8p] -> Node Voltages1/8
  [V7p] -> Node Voltages1/7
  [I1p] -> Line Currents1/1
  [V6p] -> Node Voltages1/6
  [V3p] -> Node Voltages1/3
  [I8p] -> Line Currents1/8
  [V2p] -> Node Voltages1/2
  [I6p] -> Line Currents1/6
  [I5p] -> Line Currents1/5
  [V1p] -> Node Voltages1/1
  connections:
  Three-Phase Source/RConn1 -- 66k/22k/LConn1
  Three-Phase Source/RConn2 -- 66k/22k/LConn2
  Three-Phase Source/RConn3 -- 66k/22k/LConn3
  Series RLC Load2/LConn1 -- Series RLC Load1/LConn1 -- Series RLC Load/LConn1
  Three-Phase Series RLC Branch1/RConn1 -- Three-Phase Series RLC Branch2/LConn1 -- Three-Phase Breaker16/LConn1 -- Three-Phase V-I Measurement11/RConn1
  Three-Phase Breaker16/LConn3 -- Three-Phase Series RLC Branch2/LConn3 -- Three-Phase V-I Measurement11/RConn3 -- Three-Phase Series RLC Branch1/RConn3
  Three-Phase Breaker16/LConn2 -- Three-Phase V-I Measurement11/RConn2 -- Three-Phase Series RLC Branch1/RConn2 -- Three-Phase Series RLC Branch2/LConn2
  Three-Phase Breaker/LConn1 -- 66k/22k/RConn1
  Three-Phase Breaker/LConn2 -- 66k/22k/RConn2
  Three-Phase Breaker/LConn3 -- 66k/22k/RConn3
  Three-Phase V-I Measurement/LConn1 -- Three-Phase Breaker/RConn3
  Three-Phase V-I Measurement/LConn2 -- Three-Phase Breaker/RConn2
  Three-Phase V-I Measurement/LConn3 -- Three-Phase Breaker/RConn1
  Three-Phase V-I Measurement/RConn3 -- Three-Phase Breaker5/LConn1 -- Three-Phase Breaker4/LConn1 -- Three-Phase Breaker1/LConn1 -- Three-Phase Breaker3/LConn1 -- Three-Phase Breaker2/LConn1 -- Frequency Measure/RConn1
  Frequency Measure/RConn2 -- Three-Phase Breaker5/LConn2 -- Three-Phase Breaker4/LConn2 -- Three-Phase Breaker1/LConn2 -- Three-Phase Breaker2/LConn2 -- Three-Phase Breaker3/LConn2 -- Three-Phase V-I Measurement/RConn2
  Three-Phase V-I Measurement/RConn1 -- Three-Phase Breaker5/LConn3 -- Three-Phase Breaker4/LConn3 -- Three-Phase Breaker1/LConn3 -- Three-Phase Breaker2/LConn3 -- Three-Phase Breaker3/LConn3 -- Frequency Measure/RConn3
  Three-Phase V-I Measurement1/RConn2 -- Three-Phase Transformer (Two Windings)/RConn2
  Three-Phase V-I Measurement1/RConn1 -- Three-Phase Transformer (Two Windings)/RConn1
  Three-Phase Transformer (Two Windings)/RConn3 -- Three-Phase V-I Measurement1/RConn3
  Three-Phase Series RLC Branch1/LConn1 -- Three-Phase Breaker2/RConn1
  Three-Phase Series RLC Branch1/LConn2 -- Three-Phase Breaker2/RConn2
  Three-Phase Series RLC Branch1/LConn3 -- Three-Phase Breaker2/RConn3
  DER_Site_1/LConn1 -- Three-Phase Breaker7/LConn1 -- Three-Phase V-I Measurement1/LConn1
  DER_Site_1/LConn2 -- Three-Phase Breaker7/LConn2 -- Three-Phase V-I Measurement1/LConn2
  DER_Site_1/LConn3 -- Three-Phase Breaker7/LConn3 -- Three-Phase V-I Measurement1/LConn3
  Three-Phase Transformer (Two Windings)1/LConn3 -- Three-Phase V-I Measurement18/LConn3 -- Series RLC Load5/RConn1
  Three-Phase Series RLC Branch3/RConn2 -- Three-Phase V-I Measurement18/RConn2 -- Three-Phase Breaker6/LConn2 -- Three-Phase Breaker17/LConn2
  Three-Phase Transformer (Two Windings)1/LConn1 -- Three-Phase V-I Measurement18/LConn1 -- Series RLC Load4/RConn1
  DER_Site_2/LConn1 -- Three-Phase V-I Measurement2/LConn1
  Three-Phase V-I Measurement2/RConn1 -- Three-Phase Transformer (Two Windings)1/RConn1
  Three-Phase Series RLC Branch3/LConn3 -- Three-Phase Breaker1/RConn3
  Three-Phase Series RLC Branch3/LConn2 -- Three-Phase Breaker1/RConn2
  DER_Site_2/LConn3 -- Three-Phase V-I Measurement2/LConn3
  Three-Phase Transformer (Two Windings)1/RConn3 -- Three-Phase V-I Measurement2/RConn3
  Three-Phase V-I Measurement2/RConn2 -- Three-Phase Transformer (Two Windings)1/RConn2
  Three-Phase Series RLC Branch3/LConn1 -- Three-Phase Breaker1/RConn1
  DER_Site_2/LConn2 -- Three-Phase V-I Measurement2/LConn2
  Three-Phase Series RLC Branch17/RConn3 -- Three-Phase V-I Measurement20/RConn3 -- Three-Phase Breaker12/LConn3 -- Three-Phase Series RLC Branch13/LConn3
  Three-Phase Series RLC Branch17/RConn2 -- Three-Phase V-I Measurement20/RConn2 -- Three-Phase Breaker12/LConn2 -- Three-Phase Series RLC Branch13/LConn2
  Three-Phase Transformer (Two Windings)2/LConn1 -- Three-Phase V-I Measurement20/LConn1 -- Series RLC Load7/RConn1
  DER_Site_3/LConn1 -- Three-Phase V-I Measurement3/LConn1
  Three-Phase V-I Measurement3/RConn1 -- Three-Phase Transformer (Two Windings)2/RConn1
  Three-Phase Series RLC Branch17/LConn3 -- Three-Phase Breaker3/RConn3
  Three-Phase Series RLC Branch17/LConn2 -- Three-Phase Breaker3/RConn2
  DER_Site_3/LConn3 -- Three-Phase V-I Measurement3/LConn3
  Three-Phase Transformer (Two Windings)2/RConn3 -- Three-Phase V-I Measurement3/RConn3
  Three-Phase V-I Measurement3/RConn2 -- Three-Phase Transformer (Two Windings)2/RConn2
  Three-Phase Series RLC Branch17/LConn1 -- Three-Phase Breaker3/RConn1
  DER_Site_3/LConn2 -- Three-Phase V-I Measurement3/LConn2
  Three-Phase Breaker18/LConn1 -- Three-Phase V-I Measurement19/RConn1 -- Three-Phase Breaker11/LConn1 -- Three-Phase Series RLC Branch14/LConn1 -- Three-Phase Series RLC Branch6/LConn1
  Three-Phase Breaker18/LConn2 -- Three-Phase V-I Measurement19/RConn2 -- Three-Phase Breaker11/LConn2 -- Three-Phase Series RLC Branch14/LConn2 -- Three-Phase Series RLC Branch6/LConn2
  Three-Phase Breaker18/LConn3 -- Three-Phase V-I Measurement19/RConn3 -- Three-Phase Breaker11/LConn3 -- Three-Phase Series RLC Branch14/LConn3 -- Three-Phase Series RLC Branch6/LConn3
  Three-Phase Series RLC Branch6/RConn2 -- Three-Phase Breaker4/RConn2
  DER_Site_4/LConn2 -- Three-Phase V-I Measurement4/LConn2
  Three-Phase Series RLC Branch6/RConn1 -- Three-Phase Breaker4/RConn1
  Three-Phase Series RLC Branch6/RConn3 -- Three-Phase Breaker4/RConn3
  Three-Phase Transformer (Two Windings)3/RConn3 -- Three-Phase V-I Measurement4/RConn3
  Three-Phase V-I Measurement4/RConn1 -- Three-Phase Transformer (Two Windings)3/RConn1
  Three-Phase V-I Measurement4/RConn2 -- Three-Phase Transformer (Two Windings)3/RConn2
  DER_Site_4/LConn3 -- Three-Phase V-I Measurement4/LConn3
  DER_Site_4/LConn1 -- Three-Phase V-I Measurement4/LConn1
  Three-Phase Series RLC Branch5/LConn1 -- Three-Phase V-I Measurement17/RConn1 -- Three-Phase Series RLC Branch4/LConn1 -- Three-Phase Breaker9/LConn1 -- Three-Phase Breaker8/LConn1
  Three-Phase Series RLC Branch4/LConn2 -- Three-Phase Series RLC Branch5/LConn2 -- Three-Phase Breaker8/LConn2 -- Three-Phase V-I Measurement17/RConn2 -- Three-Phase Breaker9/LConn2
  Three-Phase Transformer (Two Windings)4/LConn3 -- Three-Phase V-I Measurement17/LConn3 -- Series RLC Load14/RConn1
  Three-Phase Series RLC Branch5/RConn2 -- Three-Phase Breaker5/RConn2
  DER_Site_5/LConn2 -- Three-Phase V-I Measurement5/LConn2
  Three-Phase Series RLC Branch5/RConn1 -- Three-Phase Breaker5/RConn1
  Three-Phase Series RLC Branch5/RConn3 -- Three-Phase Breaker5/RConn3
  Three-Phase Transformer (Two Windings)4/RConn3 -- Three-Phase V-I Measurement5/RConn3
  Three-Phase V-I Measurement5/RConn1 -- Three-Phase Transformer (Two Windings)4/RConn1
  Three-Phase V-I Measurement5/RConn2 -- Three-Phase Transformer (Two Windings)4/RConn2
  DER_Site_5/LConn3 -- Three-Phase V-I Measurement5/LConn3
  DER_Site_5/LConn1 -- Three-Phase V-I Measurement5/LConn1
  Three-Phase Series RLC Branch4/RConn2 -- Three-Phase Breaker6/RConn2
  Three-Phase Series RLC Branch4/RConn3 -- Three-Phase Breaker6/RConn3
  Three-Phase Series RLC Branch4/RConn1 -- Three-Phase Breaker6/RConn1
  Three-Phase Series RLC Branch14/RConn1 -- Three-Phase Breaker8/RConn1
  Three-Phase Series RLC Branch14/RConn3 -- Three-Phase Breaker8/RConn3
  Three-Phase Series RLC Branch14/RConn2 -- Three-Phase Breaker8/RConn2
  Three-Phase Breaker10/LConn3 -- Three-Phase Series RLC Branch7/LConn3 -- Three-Phase V-I Measurement16/RConn3
  Three-Phase Breaker10/LConn2 -- Three-Phase Series RLC Branch7/LConn2 -- Three-Phase V-I Measurement16/RConn2
  Three-Phase Transformer (Two Windings)5/LConn1 -- Three-Phase V-I Measurement16/LConn1 -- Series RLC Load16/RConn1
  Three-Phase Transformer (Two Windings)5/RConn3 -- Three-Phase V-I Measurement6/RConn3
  Three-Phase V-I Measurement6/RConn2 -- Three-Phase Transformer (Two Windings)5/RConn2
  DER_Site_6/LConn2 -- Three-Phase V-I Measurement6/LConn2
  Three-Phase V-I Measurement6/RConn1 -- Three-Phase Transformer (Two Windings)5/RConn1
  DER_Site_6/LConn3 -- Three-Phase V-I Measurement6/LConn3
  DER_Site_6/LConn1 -- Three-Phase V-I Measurement6/LConn1
  Three-Phase Series RLC Branch15/RConn3 -- Three-Phase V-I Measurement15/RConn3 -- Three-Phase Breaker13/LConn3 -- Three-Phase Series RLC Branch8/LConn3
  Three-Phase Series RLC Branch15/RConn2 -- Three-Phase Series RLC Branch8/LConn2 -- Three-Phase V-I Measurement15/RConn2 -- Three-Phase Breaker13/LConn2
  Three-Phase Series RLC Branch15/RConn1 -- Three-Phase Series RLC Branch8/LConn1 -- Three-Phase V-I Measurement15/RConn1 -- Three-Phase Breaker13/LConn1
  Three-Phase Transformer (Two Windings)6/RConn3 -- Three-Phase V-I Measurement7/RConn3
  Three-Phase V-I Measurement7/RConn2 -- Three-Phase Transformer (Two Windings)6/RConn2
  DER_Site_7/LConn2 -- Three-Phase V-I Measurement7/LConn2
  Three-Phase V-I Measurement7/RConn1 -- Three-Phase Transformer (Two Windings)6/RConn1
  DER_Site_7/LConn3 -- Three-Phase V-I Measurement7/LConn3
  DER_Site_7/LConn1 -- Three-Phase V-I Measurement7/LConn1
  Three-Phase Series RLC Branch12/LConn3 -- Three-Phase Series RLC Branch9/LConn3 -- Three-Phase V-I Measurement14/RConn3 -- Three-Phase Series RLC Branch10/LConn3
  Three-Phase Series RLC Branch12/LConn2 -- Three-Phase V-I Measurement14/RConn2 -- Three-Phase Series RLC Branch10/LConn2 -- Three-Phase Series RLC Branch9/LConn2
  Series RLC Load22/RConn1 -- Three-Phase Transformer (Two Windings)7/LConn1 -- Three-Phase V-I Measurement14/LConn1
  Three-Phase Transformer (Two Windings)7/RConn3 -- Three-Phase V-I Measurement8/RConn3
  Three-Phase V-I Measurement8/RConn2 -- Three-Phase Transformer (Two Windings)7/RConn2
  DER_Site_8/LConn2 -- Three-Phase V-I Measurement8/LConn2
  Three-Phase V-I Measurement8/RConn1 -- Three-Phase Transformer (Two Windings)7/RConn1
  DER_Site_8/LConn3 -- Three-Phase V-I Measurement8/LConn3
  DER_Site_8/LConn1 -- Three-Phase V-I Measurement8/LConn1
  Three-Phase Breaker14/LConn3 -- Three-Phase V-I Measurement13/RConn3 -- Three-Phase Series RLC Branch11/LConn3
  Three-Phase Breaker14/LConn2 -- Three-Phase V-I Measurement13/RConn2 -- Three-Phase Series RLC Branch11/LConn2
  Three-Phase Transformer (Two Windings)8/LConn1 -- Series RLC Load26/RConn1 -- Three-Phase V-I Measurement13/LConn1
  Three-Phase Transformer (Two Windings)8/RConn3 -- Three-Phase V-I Measurement9/RConn3
  Three-Phase V-I Measurement9/RConn2 -- Three-Phase Transformer (Two Windings)8/RConn2
  DER_Site_9/LConn2 -- Three-Phase V-I Measurement9/LConn2
  Three-Phase V-I Measurement9/RConn1 -- Three-Phase Transformer (Two Windings)8/RConn1
  DER_Site_9/LConn3 -- Three-Phase V-I Measurement9/LConn3
  DER_Site_9/LConn1 -- Three-Phase V-I Measurement9/LConn1
  Series RLC Load27/RConn1 -- Three-Phase Transformer (Two Windings)9/LConn2 -- Three-Phase V-I Measurement12/LConn2
  Three-Phase Transformer (Two Windings)9/LConn3 -- Three-Phase V-I Measurement12/LConn3 -- Series RLC Load29/RConn1
  Three-Phase Transformer (Two Windings)9/LConn1 -- Three-Phase V-I Measurement12/LConn1 -- Series RLC Load28/RConn1
  Three-Phase V-I Measurement10/RConn1 -- Three-Phase Transformer (Two Windings)9/RConn1
  Three-Phase Transformer (Two Windings)9/RConn3 -- Three-Phase V-I Measurement10/RConn3
  DER_Site_10/LConn2 -- Three-Phase V-I Measurement10/LConn2
  Three-Phase V-I Measurement10/RConn2 -- Three-Phase Transformer (Two Windings)9/RConn2
  DER_Site_10/LConn1 -- Three-Phase V-I Measurement10/LConn1
  DER_Site_10/LConn3 -- Three-Phase V-I Measurement10/LConn3
  Three-Phase Series RLC Branch7/RConn2 -- Three-Phase Breaker9/RConn2
  Three-Phase Series RLC Branch7/RConn1 -- Three-Phase Breaker9/RConn1
  Three-Phase Series RLC Branch7/RConn3 -- Three-Phase Breaker9/RConn3
  Three-Phase Breaker11/RConn1 -- Three-Phase Series RLC Branch8/RConn1
  Three-Phase Breaker11/RConn2 -- Three-Phase Series RLC Branch8/RConn2
  Three-Phase Breaker11/RConn3 -- Three-Phase Series RLC Branch8/RConn3
  Three-Phase Series RLC Branch9/RConn1 -- Three-Phase Breaker12/RConn1
  Three-Phase Series RLC Branch9/RConn2 -- Three-Phase Breaker12/RConn2
  Three-Phase Series RLC Branch9/RConn3 -- Three-Phase Breaker12/RConn3
  Three-Phase Series RLC Branch12/RConn1 -- Three-Phase Breaker13/RConn1
  Three-Phase Series RLC Branch12/RConn2 -- Three-Phase Breaker13/RConn2
  Three-Phase Series RLC Branch12/RConn3 -- Three-Phase Breaker13/RConn3
  Three-Phase Series RLC Branch10/RConn1 -- Three-Phase Breaker14/RConn1
  Three-Phase Series RLC Branch10/RConn3 -- Three-Phase Breaker14/RConn3
  Three-Phase Series RLC Branch10/RConn2 -- Three-Phase Breaker14/RConn2
  Three-Phase Series RLC Branch11/RConn1 -- Three-Phase Breaker15/RConn1
  Three-Phase Series RLC Branch11/RConn3 -- Three-Phase Breaker15/RConn3
  Three-Phase Series RLC Branch11/RConn2 -- Three-Phase Breaker15/RConn2
  Three-Phase Series RLC Branch16/RConn1 -- Three-Phase Breaker16/RConn1
  Three-Phase Series RLC Branch16/RConn2 -- Three-Phase Breaker16/RConn2
  Three-Phase Series RLC Branch16/RConn3 -- Three-Phase Breaker16/RConn3
  Three-Phase Series RLC Branch2/RConn3 -- Three-Phase Breaker17/RConn3
  Three-Phase Series RLC Branch2/RConn1 -- Three-Phase Breaker17/RConn1
  Three-Phase Series RLC Branch2/RConn2 -- Three-Phase Breaker17/RConn2
  Three-Phase Series RLC Branch13/RConn1 -- Three-Phase Breaker18/RConn1
  Three-Phase Series RLC Branch13/RConn2 -- Three-Phase Breaker18/RConn2
  Three-Phase Series RLC Branch13/RConn3 -- Three-Phase Breaker18/RConn3
  Three-Phase Series RLC Branch15/LConn1 -- Three-Phase Breaker10/RConn1
  Three-Phase Breaker10/RConn2 -- Three-Phase Series RLC Branch15/LConn2
  Three-Phase Series RLC Branch15/LConn3 -- Three-Phase Breaker10/RConn3
  Three-Phase Breaker7/RConn1 -- DER_BESS1/RConn1
  DER_BESS1/RConn2 -- Three-Phase Breaker7/RConn2
  DER_BESS1/RConn3 -- Three-Phase Breaker7/RConn3
  Series RLC Load27/LConn1 -- Series RLC Load29/LConn1 -- Series RLC Load28/LConn1
  Series RLC Load24/LConn1 -- Series RLC Load26/LConn1 -- Series RLC Load25/LConn1
  Series RLC Load21/LConn1 -- Series RLC Load23/LConn1 -- Series RLC Load22/LConn1
  Series RLC Load6/LConn1 -- Series RLC Load8/LConn1 -- Series RLC Load7/LConn1
  Series RLC Load18/LConn1 -- Series RLC Load20/LConn1 -- Series RLC Load19/LConn1
  Series RLC Load9/LConn1 -- Series RLC Load11/LConn1 -- Series RLC Load10/LConn1
  Series RLC Load12/LConn1 -- Series RLC Load14/LConn1 -- Series RLC Load13/LConn1
  Series RLC Load15/LConn1 -- Series RLC Load17/LConn1 -- Series RLC Load16/LConn1
  Series RLC Load3/LConn1 -- Series RLC Load5/LConn1 -- Series RLC Load4/LConn1
  Three-Phase Transformer (Two Windings)/LConn3 -- Three-Phase V-I Measurement11/LConn3 -- Series RLC Load2/RConn1
  Three-Phase Transformer (Two Windings)/LConn1 -- Three-Phase V-I Measurement11/LConn1 -- Series RLC Load1/RConn1
  Three-Phase Transformer (Two Windings)/LConn2 -- Three-Phase V-I Measurement11/LConn2 -- Series RLC Load/RConn1
  Three-Phase V-I Measurement12/RConn1 -- Three-Phase Series RLC Branch16/LConn1 -- Three-Phase Breaker15/LConn1
  Three-Phase V-I Measurement12/RConn2 -- Three-Phase Series RLC Branch16/LConn2 -- Three-Phase Breaker15/LConn2
  Three-Phase V-I Measurement12/RConn3 -- Three-Phase Series RLC Branch16/LConn3 -- Three-Phase Breaker15/LConn3
  Three-Phase Transformer (Two Windings)8/LConn2 -- Series RLC Load24/RConn1 -- Three-Phase V-I Measurement13/LConn2
  Three-Phase Transformer (Two Windings)8/LConn3 -- Series RLC Load25/RConn1 -- Three-Phase V-I Measurement13/LConn3
  Three-Phase V-I Measurement13/RConn1 -- Three-Phase Series RLC Branch11/LConn1 -- Three-Phase Breaker14/LConn1
  Three-Phase Series RLC Branch12/LConn1 -- Three-Phase V-I Measurement14/RConn1 -- Three-Phase Series RLC Branch10/LConn1 -- Three-Phase Series RLC Branch9/LConn1
  Series RLC Load23/RConn1 -- Three-Phase Transformer (Two Windings)7/LConn3 -- Three-Phase V-I Measurement14/LConn3
  Series RLC Load21/RConn1 -- Three-Phase Transformer (Two Windings)7/LConn2 -- Three-Phase V-I Measurement14/LConn2
  Series RLC Load18/RConn1 -- Three-Phase Transformer (Two Windings)6/LConn2 -- Three-Phase V-I Measurement15/LConn2
  Three-Phase Transformer (Two Windings)6/LConn1 -- Three-Phase V-I Measurement15/LConn1 -- Series RLC Load19/RConn1
  Three-Phase Transformer (Two Windings)6/LConn3 -- Three-Phase V-I Measurement15/LConn3 -- Series RLC Load20/RConn1
  Three-Phase Breaker10/LConn1 -- Three-Phase Series RLC Branch7/LConn1 -- Three-Phase V-I Measurement16/RConn1
  Three-Phase Transformer (Two Windings)5/LConn2 -- Three-Phase V-I Measurement16/LConn2 -- Series RLC Load15/RConn1
  Three-Phase Transformer (Two Windings)5/LConn3 -- Three-Phase V-I Measurement16/LConn3 -- Series RLC Load17/RConn1
  Three-Phase Transformer (Two Windings)4/LConn2 -- Three-Phase V-I Measurement17/LConn2 -- Series RLC Load12/RConn1
  Three-Phase Transformer (Two Windings)4/LConn1 -- Three-Phase V-I Measurement17/LConn1 -- Series RLC Load13/RConn1
  Three-Phase Series RLC Branch4/LConn3 -- Three-Phase Series RLC Branch5/LConn3 -- Three-Phase V-I Measurement17/RConn3 -- Three-Phase Breaker8/LConn3 -- Three-Phase Breaker9/LConn3
  Three-Phase Series RLC Branch3/RConn3 -- Three-Phase V-I Measurement18/RConn3 -- Three-Phase Breaker6/LConn3 -- Three-Phase Breaker17/LConn3
  Three-Phase Transformer (Two Windings)1/LConn2 -- Three-Phase V-I Measurement18/LConn2 -- Series RLC Load3/RConn1
  Three-Phase Series RLC Branch3/RConn1 -- Three-Phase Breaker17/LConn1 -- Three-Phase V-I Measurement18/RConn1 -- Three-Phase Breaker6/LConn1
  Three-Phase Transformer (Two Windings)3/LConn1 -- Three-Phase V-I Measurement19/LConn1 -- Series RLC Load10/RConn1
  Three-Phase Transformer (Two Windings)3/LConn3 -- Three-Phase V-I Measurement19/LConn3 -- Series RLC Load11/RConn1
  Series RLC Load9/RConn1 -- Three-Phase Transformer (Two Windings)3/LConn2 -- Three-Phase V-I Measurement19/LConn2
  Three-Phase Series RLC Branch13/LConn1 -- Three-Phase Breaker12/LConn1 -- Three-Phase Series RLC Branch17/RConn1 -- Three-Phase V-I Measurement20/RConn1
  Three-Phase Transformer (Two Windings)2/LConn2 -- Three-Phase V-I Measurement20/LConn2 -- Series RLC Load6/RConn1
  Three-Phase Transformer (Two Windings)2/LConn3 -- Three-Phase V-I Measurement20/LConn3 -- Series RLC Load8/RConn1
